simulink model "boucle_ouverte"  (R2014a)
settings: Solver=VariableStepAuto  StartTime=0.0  StopTime=10  MaxStep=0.01  RelTol=1e-3
undefined symbols (not defined in the file): alpha, beta, k, to
settings Model: Creator=12210406  LastModifiedBy=UTILISATEUR
settings DataIOCC: LimitDataPoints=off  SaveFormat=Dataset
settings OptimizationCC: LifeSpan=auto  SimCompilerOptimization=off
settings DebuggingCC: MergeDetectMultiDrivingBlocksExec=error  SolverPrmCheckMsg=none  FcnCallInpInsideContextMsg=error  FrameProcessingCompatibilityMsg=error  LibraryContextMissingDiagnostic=warning  SFUnexpectedBacktrackingDiag=error  SFNoUnconditionalDefaultTransitionDiag=error
settings HardwareCC: ProdBitPerPointer=64  ProdLargestAtomicFloat=Float  ProdIntDivRoundTo=Zero  ProdEndianess=LittleEndian  ProdWordSize=64  ProdHWDeviceType=Intel->x86-64 (Windows64)
settings ModelReferenceCC: PropagateSignalLabelsOutOfModel=on
settings SFSimCC: SimUseLocalCustomCode=on
settings RTWCC: RTWUseLocalCustomCode=on  RTWCompilerOptimization=off
settings GRTTargetCC: TargetLangStandard=C99 (ISO)  GeneratePreprocessorConditionals=Use local settings

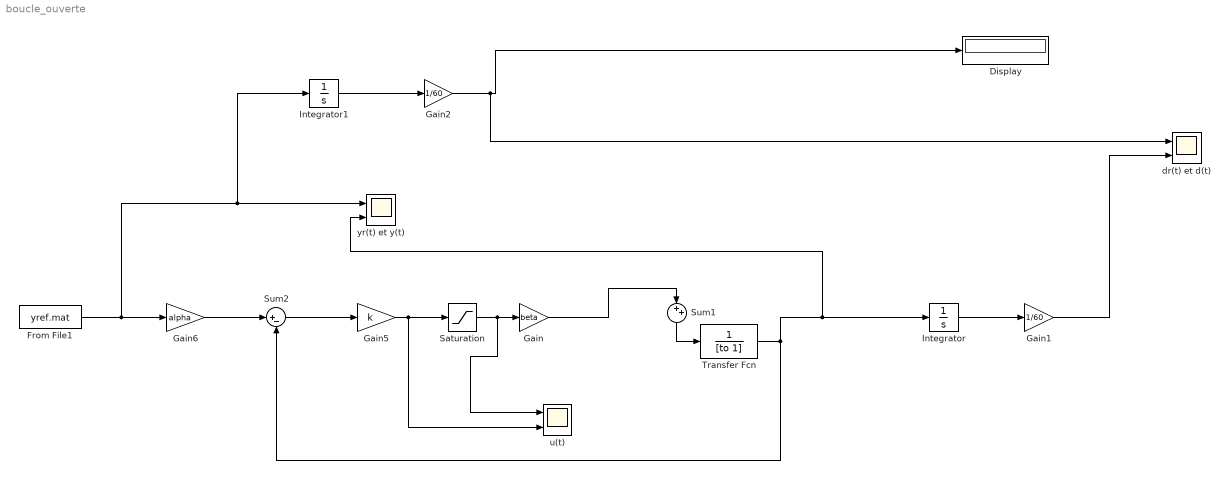
== system boucle_ouverte ==
  Display : Display
  From File1 : FromFile  FileName=yref.mat  SampleTime=0
  Gain : Gain  Gain=beta
  Gain1 : Gain  Gain=1/60
  Gain2 : Gain  Gain=1/60
  Gain5 : Gain  Gain=k
  Gain6 : Gain  Gain=alpha
  Integrator : Integrator  UpperSaturationLimit=t  LowerSaturationLimit=0
  Integrator1 : Integrator  UpperSaturationLimit=t  LowerSaturationLimit=0
  Saturation : Saturate  UpperLimit=100  LowerLimit=-50
  Sum1 : Sum  Inputs=|++
  Sum2 : Sum  Inputs=|+-
  Transfer Fcn : TransferFcn  Denominator=[to 1]
  dr(t) et d(t) : Scope  NumInputPorts=2
      settings: YMin=-5~-5  YMax=5~5
  u(t) : Scope  NumInputPorts=2
  yr(t) et y(t) : Scope  NumInputPorts=2
      settings: SaveName=ScopeData5
  wires:
  Transfer Fcn/1 -> yr(t) et y(t)/2, Integrator/1, Sum2/2
  Integrator/1 -> Gain1/1
  Saturation/1 -> u(t)/1, Gain/1
  Gain6/1 -> Sum2/1
  Sum2/1 -> Gain5/1
  Gain5/1 -> u(t)/2, Saturation/1
  Sum1/1 -> Transfer Fcn/1
  Integrator1/1 -> Gain2/1
  Gain2/1 -> dr(t) et d(t)/1, Display/1
  Gain/1 -> Sum1/1
  From File1/1 -> Integrator1/1, yr(t) et y(t)/1, Gain6/1
  Gain1/1 -> dr(t) et d(t)/2
